simulink model "overall_model"  (R2015a)
settings: Solver=ode45  StartTime=0.0  StopTime=10.0  RelTol=1e-3
libraries: fuzblock x2
settings Model: Creator=BML  LastModifiedBy=BML

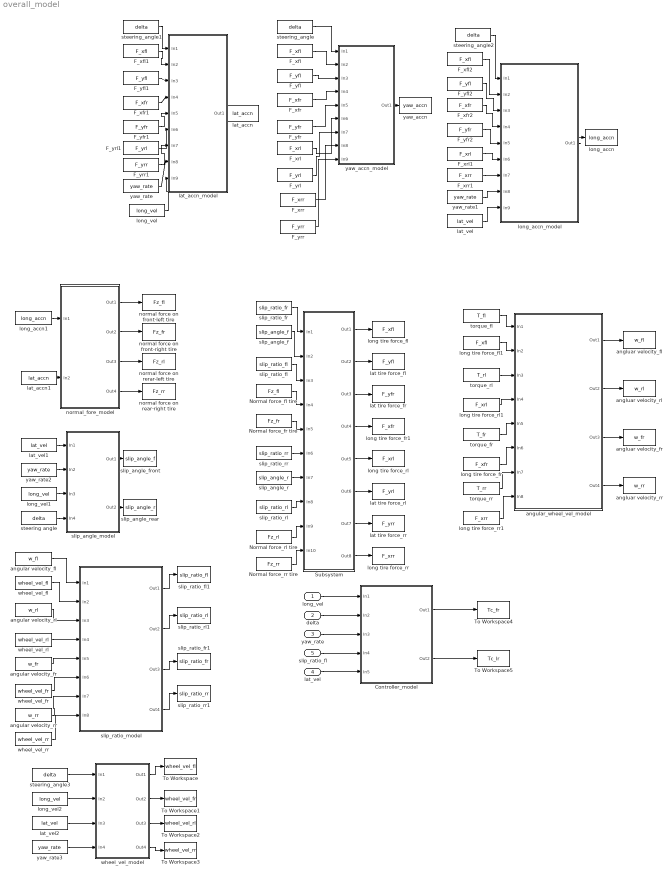
== system overall_model ==
  "  long_vel  " : Inport
  "  delta " : Inport  Port=2
  "  yaw_rate " : Inport  Port=3
  "  lat_vel" : Inport  Port=4
  " slip_ratio_fl  " : Inport  Port=5
  Controller_model : Subsystem
  F_xfl : FromWorkspace  VariableName=F_xfl  SampleTime=0
  F_xfl1 : FromWorkspace  VariableName=F_xfl  SampleTime=0
  F_xfl2 : FromWorkspace  VariableName=F_xfl  SampleTime=0
  F_xfr : FromWorkspace  VariableName=F_xfr  SampleTime=0
  F_xfr1 : FromWorkspace  VariableName=F_xfr  SampleTime=0
  F_xfr2 : FromWorkspace  VariableName=F_xfr  SampleTime=0
  F_xrl : FromWorkspace  VariableName=F_xrl  SampleTime=0
  F_xrl1 : FromWorkspace  VariableName=F_xrl  SampleTime=0
  F_xrr : FromWorkspace  VariableName=F_xrr  SampleTime=0
  F_xrr1 : FromWorkspace  VariableName=F_xrr  SampleTime=0
  F_yfl : FromWorkspace  VariableName=F_yfl  SampleTime=0
  F_yfl1 : FromWorkspace  VariableName=F_yfl  SampleTime=0
  F_yfl2 : FromWorkspace  VariableName=F_yfl  SampleTime=0
  F_yfr : FromWorkspace  VariableName=F_yfr  SampleTime=0
  F_yfr1 : FromWorkspace  VariableName=F_yfr  SampleTime=0
  F_yfr2 : FromWorkspace  VariableName=F_yfr  SampleTime=0
  F_yrl : FromWorkspace  VariableName=F_yrl  SampleTime=0
  F_yrl1 : FromWorkspace  VariableName=F_yrl  SampleTime=0
  F_yrr : FromWorkspace  VariableName=F_yrr  SampleTime=0
  F_yrr1 : FromWorkspace  VariableName=F_yrr  SampleTime=0
  Normal force_fl tire : FromWorkspace  VariableName=Fz_fl  SampleTime=0
  Normal force_fr tire : FromWorkspace  VariableName=Fz_fr  SampleTime=0
  Normal force_rl tire : FromWorkspace  VariableName=Fz_rl  SampleTime=0
  Normal force_rr tire : FromWorkspace  VariableName=Fz_rr  SampleTime=0
  Subsystem : Subsystem
  To Workspace : ToWorkspace  VariableName=wheel_vel_fl  SaveFormat=Timeseries  SampleTime=-1
  To Workspace1 : ToWorkspace  VariableName=wheel_vel_fr  SaveFormat=Timeseries  SampleTime=-1
  To Workspace2 : ToWorkspace  VariableName=wheel_vel_rl  SaveFormat=Timeseries  SampleTime=-1
  To Workspace3 : ToWorkspace  VariableName=wheel_vel_rr  SaveFormat=Timeseries  SampleTime=-1
  To Workspace4 : ToWorkspace  VariableName=Tc_fr  SaveFormat=Timeseries  SampleTime=-1
  To Workspace5 : ToWorkspace  VariableName=Tc_lr  SaveFormat=Timeseries  SampleTime=-1
  angluar velocity_fl : ToWorkspace  VariableName=w_fl  SaveFormat=Timeseries  SampleTime=-1
  angluar velocity_fr : ToWorkspace  VariableName=w_fr  SaveFormat=Timeseries  SampleTime=-1
  angluar velocity_rl : ToWorkspace  VariableName=w_rl  SaveFormat=Timeseries  SampleTime=-1
  angluar velocity_rr : ToWorkspace  VariableName=w_rr  SaveFormat=Timeseries  SampleTime=-1
  angular velocity_fl : FromWorkspace  VariableName=w_fl  SampleTime=0
  angular velocity_fr : FromWorkspace  VariableName=w_fr  SampleTime=0
  angular velocity_rl : FromWorkspace  VariableName=w_rl  SampleTime=0
  angular velocity_rr : FromWorkspace  VariableName=w_rr  SampleTime=0
  angular_wheel_vel_model : Subsystem
  lat tire force_fl : ToWorkspace  VariableName=F_yfl  SaveFormat=Timeseries  SampleTime=-1
  lat tire force_fr : ToWorkspace  VariableName=F_yfr  SaveFormat=Timeseries  SampleTime=-1
  lat tire force_rl : ToWorkspace  VariableName=F_yrl  SaveFormat=Timeseries  SampleTime=-1
  lat tire force_rr : ToWorkspace  VariableName=F_yrr  SaveFormat=Timeseries  SampleTime=-1
  lat_accn : ToWorkspace  VariableName=lat_accn  SaveFormat=Timeseries  SampleTime=-1
  lat_accn1 : FromWorkspace  VariableName=lat_accn  SampleTime=0
  lat_accn_model : Subsystem
  lat_vel : FromWorkspace  VariableName=lat_vel  SampleTime=0
  lat_vel1 : FromWorkspace  VariableName=lat_vel  SampleTime=0
  lat_vel2 : FromWorkspace  VariableName=lat_vel  SampleTime=0
  long tire force_fl : ToWorkspace  VariableName=F_xfl  SaveFormat=Timeseries  SampleTime=-1
  long tire force_fl1 : FromWorkspace  VariableName=F_xfl  SampleTime=0
  long tire force_fr : FromWorkspace  VariableName=F_xfr  SampleTime=0
  long tire force_fr1 : ToWorkspace  VariableName=F_xfr  SaveFormat=Timeseries  SampleTime=-1
  long tire force_rl : ToWorkspace  VariableName=F_xrl  SaveFormat=Timeseries  SampleTime=-1
  long tire force_rl1 : FromWorkspace  VariableName=F_xrl  SampleTime=0
  long tire force_rr : ToWorkspace  VariableName=F_xrr  SaveFormat=Timeseries  SampleTime=-1
  long tire force_rr1 : FromWorkspace  VariableName=F_xrr  SampleTime=0
  long_accn : ToWorkspace  VariableName=long_accn  SaveFormat=Timeseries  SampleTime=-1
  long_accn1 : FromWorkspace  VariableName=long_accn  SampleTime=0
  long_accn_model : Subsystem
  long_vel : FromWorkspace  VariableName=long_vel  SampleTime=0
  long_vel1 : FromWorkspace  VariableName=long_vel  SampleTime=0
  long_vel2 : FromWorkspace  VariableName=long_vel  SampleTime=0
  normal force on front-left tire : ToWorkspace  VariableName=Fz_fl  SaveFormat=Timeseries  SampleTime=-1
  normal force on front-right tire : ToWorkspace  VariableName=Fz_fr  SaveFormat=Timeseries  SampleTime=-1
  normal force on rear-right tire : ToWorkspace  VariableName=Fz_rr  SaveFormat=Timeseries  SampleTime=-1
  normal force on rerar-left tire : ToWorkspace  VariableName=Fz_rl  SaveFormat=Timeseries  SampleTime=-1
  normal_fore_model : Subsystem
  slip_angle_f : FromWorkspace  VariableName=slip_angle_f  SampleTime=0
  slip_angle_front : ToWorkspace  VariableName=slip_angle_f  SaveFormat=Timeseries  SampleTime=-1
  slip_angle_model : Subsystem
  slip_angle_r : FromWorkspace  VariableName=slip_angle_r  SampleTime=0
  slip_angle_rear : ToWorkspace  VariableName=slip_angle_r  SaveFormat=Timeseries  SampleTime=-1
  slip_ratio_fl : FromWorkspace  VariableName=slip_ratio_fl  SampleTime=0
  slip_ratio_fl1 : ToWorkspace  VariableName=slip_ratio_fl  SaveFormat=Timeseries  SampleTime=-1
  slip_ratio_fr : FromWorkspace  VariableName=slip_ratio_fr  SampleTime=0
  slip_ratio_fr1 : ToWorkspace  VariableName=slip_ratio_fr  SaveFormat=Timeseries  SampleTime=-1
  slip_ratio_model : Subsystem
  slip_ratio_rl : FromWorkspace  VariableName=slip_ratio_rl  SampleTime=0
  slip_ratio_rl1 : ToWorkspace  VariableName=slip_ratio_rl  SaveFormat=Timeseries  SampleTime=-1
  slip_ratio_rr : FromWorkspace  VariableName=slip_ratio_rr  SampleTime=0
  slip_ratio_rr1 : ToWorkspace  VariableName=slip_ratio_rr  SaveFormat=Timeseries  SampleTime=-1
  steering angle : FromWorkspace  VariableName=delta  SampleTime=0
  steering_angle{,1..3} (4 alike) : FromWorkspace  VariableName=delta  SampleTime=0
  torque_fl : FromWorkspace  VariableName=T_fl  SampleTime=0
  torque_fr : FromWorkspace  VariableName=T_fr  SampleTime=0
  torque_rl : FromWorkspace  VariableName=T_rl  SampleTime=0
  torque_rr : FromWorkspace  VariableName=T_rr  SampleTime=0
  wheel_vel_fl : FromWorkspace  VariableName=wheel_vel_fl  SampleTime=0
  wheel_vel_fr : FromWorkspace  VariableName=wheel_vel_fr  SampleTime=0
  wheel_vel_model : Subsystem
  wheel_vel_rl : FromWorkspace  VariableName=wheel_vel_rl  SampleTime=0
  wheel_vel_rr : FromWorkspace  VariableName=wheel_vel_rr  SampleTime=0
  yaw_accn : ToWorkspace  VariableName=yaw_accn  SaveFormat=Timeseries  SampleTime=-1
  yaw_accn_model : Subsystem
  yaw_rate{,1..3} (4 alike) : FromWorkspace  VariableName=yaw_rate  SampleTime=0
  wires:
  steering_angle/1 -> yaw_accn_model/1(In1)
  F_xfl/1 -> yaw_accn_model/2(In2)
  F_yfl/1 -> yaw_accn_model/3(In3)
  F_xfr/1 -> yaw_accn_model/4(In4)
  F_yfr/1 -> yaw_accn_model/5(In5)
  F_xrl/1 -> yaw_accn_model/6(In6)
  F_yrl/1 -> yaw_accn_model/7(In7)
  F_xrr/1 -> yaw_accn_model/8(In8)
  F_yrr/1 -> yaw_accn_model/9(In9)
  yaw_accn_model/1(Out1) -> yaw_accn/1
  steering_angle1/1 -> lat_accn_model/1(In1)
  F_xfl1/1 -> lat_accn_model/2(In2)
  F_yfl1/1 -> lat_accn_model/3(In3)
  F_xfr1/1 -> lat_accn_model/4(In4)
  F_yfr1/1 -> lat_accn_model/5(In5)
  F_yrl1/1 -> lat_accn_model/6(In6)
  F_yrr1/1 -> lat_accn_model/7(In7)
  yaw_rate/1 -> lat_accn_model/8(In8)
  long_vel/1 -> lat_accn_model/9(In9)
  lat_accn_model/1(Out1) -> lat_accn/1
  steering_angle2/1 -> long_accn_model/1(In1)
  F_xfl2/1 -> long_accn_model/2(In2)
  F_yfl2/1 -> long_accn_model/3(In3)
  F_xfr2/1 -> long_accn_model/4(In4)
  F_yfr2/1 -> long_accn_model/5(In5)
  F_xrl1/1 -> long_accn_model/6(In6)
  F_xrr1/1 -> long_accn_model/7(In7)
  yaw_rate1/1 -> long_accn_model/8(In8)
  lat_vel/1 -> long_accn_model/9(In9)
  long_accn_model/1(Out1) -> long_accn/1
  long_accn1/1 -> normal_fore_model/1(In1)
  lat_accn1/1 -> normal_fore_model/2(In2)
  normal_fore_model/1(Out1) -> normal force on front-left tire/1
  normal_fore_model/2(Out2) -> normal force on front-right tire/1
  normal_fore_model/3(Out3) -> normal force on rerar-left tire/1
  normal_fore_model/4(Out4) -> normal force on rear-right tire/1
  lat_vel1/1 -> slip_angle_model/1(In1)
  yaw_rate2/1 -> slip_angle_model/2(In2)
  long_vel1/1 -> slip_angle_model/3(In3)
  steering angle/1 -> slip_angle_model/4(In4)
  slip_angle_model/1(Out1) -> slip_angle_front/1
  slip_angle_model/2(Out2) -> slip_angle_rear/1
  angular velocity_fl/1 -> slip_ratio_model/1(In1)
  wheel_vel_fl/1 -> slip_ratio_model/2(In2)
  angular velocity_rl/1 -> slip_ratio_model/3(In3)
  wheel_vel_rl/1 -> slip_ratio_model/4(In4)
  angular velocity_fr/1 -> slip_ratio_model/5(In5)
  wheel_vel_fr/1 -> slip_ratio_model/6(In6)
  angular velocity_rr/1 -> slip_ratio_model/7(In7)
  wheel_vel_rr/1 -> slip_ratio_model/8(In8)
  slip_ratio_model/1(Out1) -> slip_ratio_fl1/1
  slip_ratio_model/2(Out2) -> slip_ratio_rl1/1
  slip_ratio_model/3(Out3) -> slip_ratio_fr1/1
  slip_ratio_model/4(Out4) -> slip_ratio_rr1/1
  steering_angle3/1 -> wheel_vel_model/1(In1)
  long_vel2/1 -> wheel_vel_model/2(In2)
  lat_vel2/1 -> wheel_vel_model/3(In3)
  yaw_rate3/1 -> wheel_vel_model/4(In4)
  wheel_vel_model/1(Out1) -> To Workspace/1
  wheel_vel_model/2(Out2) -> To Workspace1/1
  wheel_vel_model/3(Out3) -> To Workspace2/1
  wheel_vel_model/4(Out4) -> To Workspace3/1
  torque_fl/1 -> angular_wheel_vel_model/1(In1)
  long tire force_fl1/1 -> angular_wheel_vel_model/2(In2)
  torque_rl/1 -> angular_wheel_vel_model/3(In3)
  long tire force_rl1/1 -> angular_wheel_vel_model/4(In4)
  torque_fr/1 -> angular_wheel_vel_model/5(In5)
  long tire force_fr/1 -> angular_wheel_vel_model/6(In6)
  torque_rr/1 -> angular_wheel_vel_model/7(In7)
  long tire force_rr1/1 -> angular_wheel_vel_model/8(In8)
  angular_wheel_vel_model/1(Out1) -> angluar velocity_fl/1
  angular_wheel_vel_model/2(Out2) -> angluar velocity_rl/1
  angular_wheel_vel_model/3(Out3) -> angluar velocity_fr/1
  angular_wheel_vel_model/4(Out4) -> angluar velocity_rr/1
  "  long_vel  "/1 -> Controller_model/1(In1)
  "  delta "/1 -> Controller_model/2(In2)
  "  yaw_rate "/1 -> Controller_model/3(In3)
  " slip_ratio_fl  "/1 -> Controller_model/4(In4)
  "  lat_vel"/1 -> Controller_model/5(In5)
  Controller_model/1(Out1) -> To Workspace4/1
  Controller_model/2(Out2) -> To Workspace5/1
  slip_ratio_fr/1 -> Subsystem/1(In1)
  slip_angle_f/1 -> Subsystem/2(In2)
  slip_ratio_fl/1 -> Subsystem/3(In3)
  Normal force_fl tire/1 -> Subsystem/4(In4)
  Normal force_fr tire/1 -> Subsystem/5(In5)
  slip_ratio_rr/1 -> Subsystem/6(In6)
  slip_angle_r/1 -> Subsystem/7(In7)
  slip_ratio_rl/1 -> Subsystem/8(In8)
  Normal force_rl tire/1 -> Subsystem/9(In9)
  Normal force_rr tire/1 -> Subsystem/10(In10)
  Subsystem/1(Out1) -> long tire force_fl/1
  Subsystem/2(Out2) -> lat tire force_fl/1
  Subsystem/3(Out3) -> lat tire force_fr/1
  Subsystem/4(Out4) -> long tire force_fr1/1
  Subsystem/5(Out5) -> long tire force_rl/1
  Subsystem/6(Out6) -> lat tire force_rl/1
  Subsystem/7(Out7) -> lat tire force_rr/1
  Subsystem/8(Out8) -> long tire force_rr/1

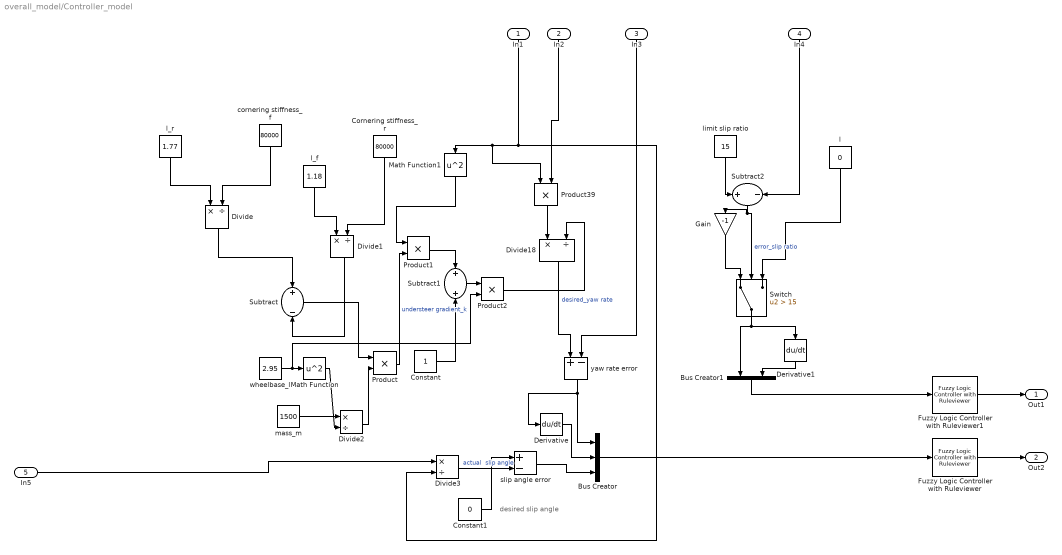
== system overall_model/Controller_model ==
  note: desired
      | slip angle
  In1 : Inport
  In2 : Inport  Port=2
  In3 : Inport  Port=3
  In4 : Inport  Port=4
  In5 : Inport  Port=5
  Bus Creator : BusCreator  Inputs=3
  Bus Creator1 : BusCreator  Inputs=2
  Constant : Constant
  Constant1 : Constant  Value=0
  "Cornering stiffness_r " : Constant  Value=80000
  Derivative : Derivative
  Derivative1 : Derivative
  Divide{,1..3,18} (5 alike) : Product  Inputs=*/
  Fuzzy Logic Controller with Ruleviewer : fuzblock/Fuzzy Logic  Controller  with Ruleviewer  fismatrix=yaw_rate  Ts=2
  Fuzzy Logic Controller with Ruleviewer1 : fuzblock/Fuzzy Logic  Controller  with Ruleviewer  fismatrix=slip_ratio  Ts=2
  Gain : Gain  Gain=-1
  Math Function : Math  Operator=square  SaturateOnIntegerOverflow=on
  Math Function1 : Math  Operator=square  SaturateOnIntegerOverflow=on
  Product{,1..2,39} (4 alike) : Product
  Subtract : Sum  Inputs=+-
  Subtract1 : Sum
  Subtract2 : Sum  Inputs=+-
  Switch : Switch  Criteria=u2 > Threshold  Threshold=15
  "cornering stiffness_f " : Constant  Value=80000
  l : Constant  Value=0
  "l_f " : Constant  Value=1.18
  "l_r " : Constant  Value=1.77
  limit slip ratio : Constant  Value=15
  mass_m : Constant  Value=1500
  "slip angle error  " : Sum  Inputs=+-
  wheelbase_l : Constant  Value=2.95
  "yaw rate error   " : Sum  Inputs=+-
  Out1 : Outport
  Out2 : Outport  Port=2
  wires:
  Fuzzy Logic Controller with Ruleviewer1/1 -> Out1/1
  Divide/1 -> Subtract/1
  Subtract/1 -> Product/1
  Product/1 -> Product1/2  "understeer gradient_k"
  Constant/1 -> Subtract1/2
  Product39/1 -> Divide18/1
  Product2/1 -> Divide18/2
  In2/1 -> Product39/2
  Math Function1/1 -> Product1/1
  Subtract1/1 -> Product2/1
  In5/1 -> Divide3/1
  "l_r "/1 -> Divide/1
  Divide1/1 -> Subtract/2
  "Cornering stiffness_r "/1 -> Divide1/2
  wheelbase_l/1 -> Product2/2, Math Function/1
  mass_m/1 -> Divide2/1
  Math Function/1 -> Divide2/2
  Divide2/1 -> Product/2
  In1/1 -> Divide3/2, Math Function1/1, Product39/1
  "l_f "/1 -> Divide1/1
  "cornering stiffness_f "/1 -> Divide/2
  Product1/1 -> Subtract1/1
  Constant1/1 -> "slip angle error  "/1
  Switch/1 -> Derivative1/1, Bus Creator1/1
  In3/1 -> "yaw rate error   "/2
  Divide18/1 -> "yaw rate error   "/1  "desired_yaw rate"
  Subtract2/1 -> Switch/2, Gain/1  "error_slip ratio"
  Gain/1 -> Switch/1
  "yaw rate error   "/1 -> Bus Creator/1, Derivative/1
  limit slip ratio/1 -> Subtract2/1
  Derivative/1 -> Bus Creator/2
  Bus Creator/1 -> Fuzzy Logic Controller with Ruleviewer/1
  In4/1 -> Subtract2/2
  l/1 -> Switch/3
  Divide3/1 -> "slip angle error  "/2  "actual  slip angle"
  "slip angle error  "/1 -> Bus Creator/3
  Derivative1/1 -> Bus Creator1/2
  Bus Creator1/1 -> Fuzzy Logic Controller with Ruleviewer1/1
  Fuzzy Logic Controller with Ruleviewer/1 -> Out2/1

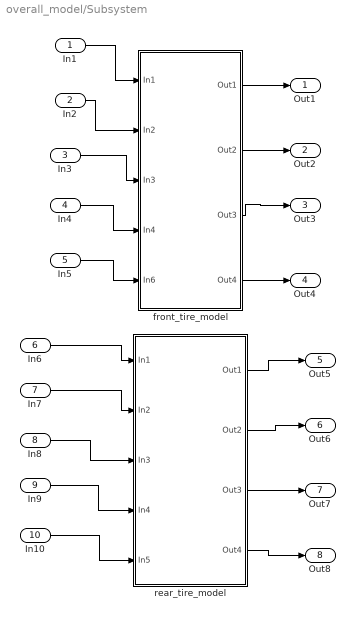
== system overall_model/Subsystem ==
  In1 : Inport
  In2 : Inport  Port=2
  In3 : Inport  Port=3
  In4 : Inport  Port=4
  In5 : Inport  Port=5
  In6 : Inport  Port=6
  In7 : Inport  Port=7
  In8 : Inport  Port=8
  In9 : Inport  Port=9
  In10 : Inport  Port=10
  front_tire_model : Subsystem
  rear_tire_model : Subsystem
  Out1 : Outport
  Out2 : Outport  Port=2
  Out3 : Outport  Port=3
  Out4 : Outport  Port=4
  Out5 : Outport  Port=5
  Out6 : Outport  Port=6
  Out7 : Outport  Port=7
  Out8 : Outport  Port=8
  wires:
  In6/1 -> rear_tire_model/1(In1)
  In7/1 -> rear_tire_model/2(In2)
  rear_tire_model/3(Out3) -> Out7/1
  In8/1 -> rear_tire_model/3(In3)
  rear_tire_model/2(Out2) -> Out6/1
  In10/1 -> rear_tire_model/5(In5)
  rear_tire_model/1(Out1) -> Out5/1
  rear_tire_model/4(Out4) -> Out8/1
  In9/1 -> rear_tire_model/4(In4)
  In2/1 -> front_tire_model/2(In2)
  In1/1 -> front_tire_model/1(In1)
  In3/1 -> front_tire_model/3(In3)
  In5/1 -> front_tire_model/5(In6)
  front_tire_model/1(Out1) -> Out1/1
  front_tire_model/3(Out3) -> Out3/1
  front_tire_model/2(Out2) -> Out2/1
  In4/1 -> front_tire_model/4(In4)
  front_tire_model/4(Out4) -> Out4/1

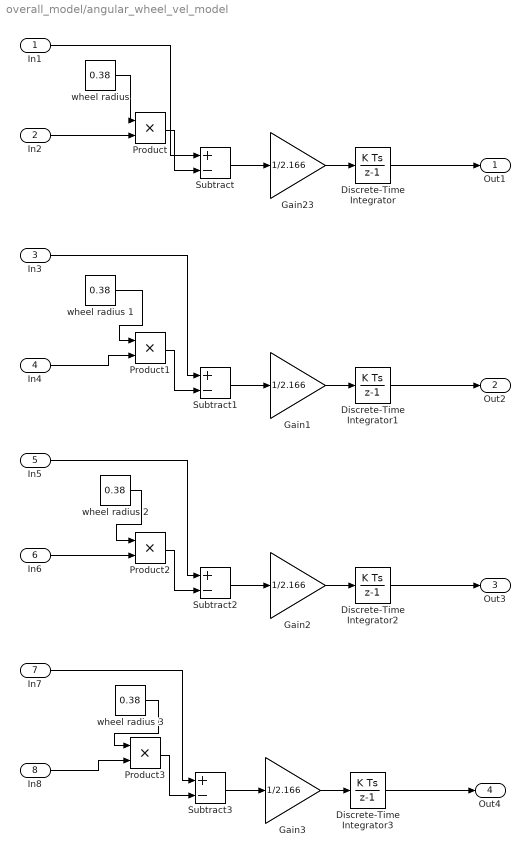
== system overall_model/angular_wheel_vel_model ==
  In1 : Inport
  In2 : Inport  Port=2
  In3 : Inport  Port=3
  In4 : Inport  Port=4
  In5 : Inport  Port=5
  In6 : Inport  Port=6
  In7 : Inport  Port=7
  In8 : Inport  Port=8
  Discrete-Time Integrator{,1..3} (4 alike) : DiscreteIntegrator  InitialConditionSetting=State (most efficient)
  Gain{1..3,23} (4 alike) : Gain  Gain=1/2.166
  Product{,1..3} (4 alike) : Product
  Subtract{,1..3} (4 alike) : Sum  Inputs=+-
  wheel radius {,1..3} (4 alike) : Constant  Value=0.38
  Out1 : Outport
  Out2 : Outport  Port=2
  Out3 : Outport  Port=3
  Out4 : Outport  Port=4
  wires:
  Gain23/1 -> Discrete-Time Integrator/1
  Discrete-Time Integrator/1 -> Out1/1
  In2/1 -> Product/2
  Product/1 -> Subtract/2
  wheel radius 1/1 -> Product1/1
  In3/1 -> Subtract1/1
  In1/1 -> Subtract/1
  Subtract/1 -> Gain23/1
  In4/1 -> Product1/2
  "wheel radius "/1 -> Product/1
  Subtract2/1 -> Gain2/1
  wheel radius 2/1 -> Product2/1
  Product1/1 -> Subtract1/2
  In8/1 -> Product3/2
  In7/1 -> Subtract3/1
  Gain3/1 -> Discrete-Time Integrator3/1
  Subtract1/1 -> Gain1/1
  Gain1/1 -> Discrete-Time Integrator1/1
  Gain2/1 -> Discrete-Time Integrator2/1
  Subtract3/1 -> Gain3/1
  Discrete-Time Integrator3/1 -> Out4/1
  wheel radius 3/1 -> Product3/1
  In6/1 -> Product2/2
  Product3/1 -> Subtract3/2
  In5/1 -> Subtract2/1
  Product2/1 -> Subtract2/2
  Discrete-Time Integrator1/1 -> Out2/1
  Discrete-Time Integrator2/1 -> Out3/1

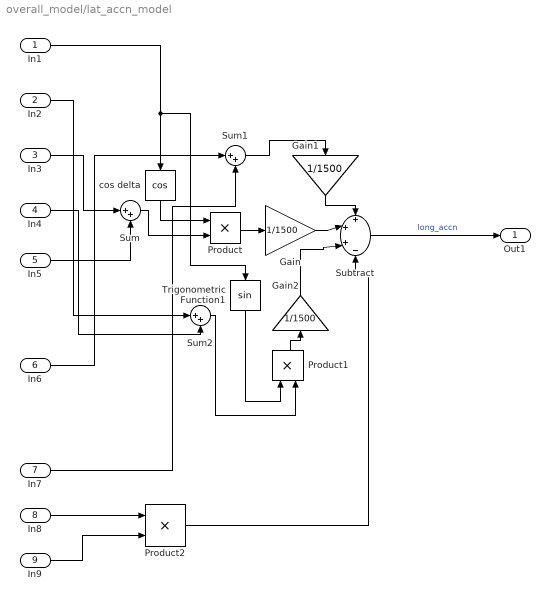
== system overall_model/lat_accn_model ==
  In1 : Inport
  In2 : Inport  Port=2
  In3 : Inport  Port=3
  In4 : Inport  Port=4
  In5 : Inport  Port=5
  In6 : Inport  Port=6
  In7 : Inport  Port=7
  In8 : Inport  Port=8
  In9 : Inport  Port=9
  Gain : Gain  Gain=1/1500
  Gain1 : Gain  Gain=1/1500
  Gain2 : Gain  Gain=1/1500
  Product : Product
  Product1 : Product
  Product2 : Product
  Subtract : Sum  Inputs=+++-
  Sum : Sum  Inputs=|++
  Sum1 : Sum  Inputs=|++
  Sum2 : Sum  Inputs=|++
  Trigonometric Function1 : Trigonometry
  cos delta : Trigonometry  Operator=cos
  Out1 : Outport
  wires:
  Gain/1 -> Subtract/2
  cos delta/1 -> Product/1
  Sum/1 -> Product/2
  Gain1/1 -> Subtract/1
  Sum1/1 -> Gain1/1
  In9/1 -> Product2/2
  Product/1 -> Gain/1
  In1/1 -> Trigonometric Function1/1, cos delta/1
  Trigonometric Function1/1 -> Product1/1
  Sum2/1 -> Product1/2
  Subtract/1 -> Out1/1  "long_accn"
  Product2/1 -> Subtract/4
  Product1/1 -> Gain2/1
  In4/1 -> Sum2/2
  In2/1 -> Sum2/1
  Gain2/1 -> Subtract/3
  In5/1 -> Sum/2
  In6/1 -> Sum1/1
  In8/1 -> Product2/1
  In3/1 -> Sum/1
  In7/1 -> Sum1/2

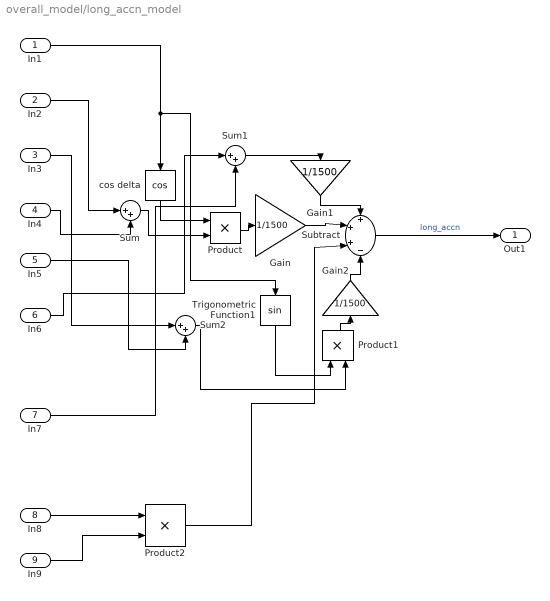
== system overall_model/long_accn_model ==
  In1 : Inport
  In2 : Inport  Port=2
  In3 : Inport  Port=3
  In4 : Inport  Port=4
  In5 : Inport  Port=5
  In6 : Inport  Port=6
  In7 : Inport  Port=7
  In8 : Inport  Port=8
  In9 : Inport  Port=9
  Gain : Gain  Gain=1/1500
  Gain1 : Gain  Gain=1/1500
  Gain2 : Gain  Gain=1/1500
  Product : Product
  Product1 : Product
  Product2 : Product
  Subtract : Sum  Inputs=+++-
  Sum : Sum  Inputs=|++
  Sum1 : Sum  Inputs=|++
  Sum2 : Sum  Inputs=|++
  Trigonometric Function1 : Trigonometry
  cos delta : Trigonometry  Operator=cos
  Out1 : Outport
  wires:
  Product2/1 -> Subtract/3
  Gain/1 -> Subtract/2
  cos delta/1 -> Product/1
  Sum/1 -> Product/2
  Product/1 -> Gain/1
  Gain1/1 -> Subtract/1
  In7/1 -> Sum1/2
  In9/1 -> Product2/2
  Sum1/1 -> Gain1/1
  In4/1 -> Sum/2
  In6/1 -> Sum1/1
  In2/1 -> Sum/1
  In3/1 -> Sum2/1
  In5/1 -> Sum2/2
  Product1/1 -> Gain2/1
  In1/1 -> Trigonometric Function1/1, cos delta/1
  Trigonometric Function1/1 -> Product1/1
  Subtract/1 -> Out1/1  "long_accn"
  Sum2/1 -> Product1/2
  Gain2/1 -> Subtract/4
  In8/1 -> Product2/1

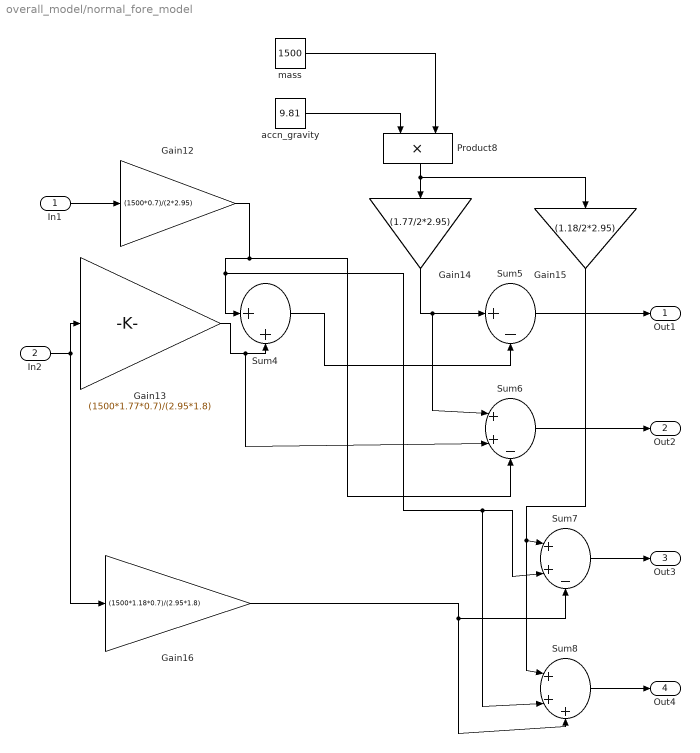
== system overall_model/normal_fore_model ==
  In1 : Inport
  In2 : Inport  Port=2
  Gain12 : Gain  Gain=(1500*0.7)/(2*2.95)
  Gain13 : Gain  Gain=(1500*1.77*0.7)/(2.95*1.8)
  Gain14 : Gain  Gain=(1.77/2*2.95)
  Gain15 : Gain  Gain=(1.18/2*2.95)
  Gain16 : Gain  Gain=(1500*1.18*0.7)/(2.95*1.8)
  Product8 : Product
  Sum4 : Sum  Inputs=|++
  Sum5 : Sum  Inputs=|+-
  Sum6 : Sum  Inputs=|++-
  Sum7 : Sum  Inputs=|++-
  Sum8 : Sum  Inputs=|+++
  "accn_gravity " : Constant  Value=9.81
  mass : Constant  Value=1500
  Out1 : Outport
  Out2 : Outport  Port=2
  Out3 : Outport  Port=3
  Out4 : Outport  Port=4
  wires:
  Gain12/1 -> Sum4/1, Sum8/2, Sum7/2, Sum6/3
  Gain15/1 -> Sum8/1, Sum7/1
  Gain16/1 -> Sum8/3, Sum7/3
  Sum7/1 -> Out3/1
  In2/1 -> Gain13/1, Gain16/1
  Gain13/1 -> Sum6/2, Sum4/2
  Sum5/1 -> Out1/1
  Sum6/1 -> Out2/1
  Sum4/1 -> Sum5/2
  In1/1 -> Gain12/1
  mass/1 -> Product8/2
  Gain14/1 -> Sum5/1, Sum6/1
  Sum8/1 -> Out4/1
  Product8/1 -> Gain14/1, Gain15/1
  "accn_gravity "/1 -> Product8/1

== system overall_model/slip_angle_model ==
  In1 : Inport
  In2 : Inport  Port=2
  In3 : Inport  Port=3
  In4 : Inport  Port=4
  Divide4 : Product  Inputs=*/
  Divide5 : Product  Inputs=*/
  Product : Product
  Product1 : Product
  Sum4 : Sum  Inputs=|++
  Sum5 : Sum  Inputs=|+-
  Sum6 : Sum  Inputs=|+-
  l_f : Constant  Value=1.18
  l_r : Constant  Value=1.77
  Out1 : Outport
  Out2 : Outport  Port=2
  wires:
  In2/1 -> Product1/2, Product/2
  In3/1 -> Divide5/2, Divide4/2
  l_f/1 -> Product/1
  In1/1 -> Sum6/2, Sum4/1
  Divide4/1 -> Sum5/2
  Product/1 -> Sum4/2
  Sum4/1 -> Divide4/1
  Divide5/1 -> Out2/1
  In4/1 -> Sum5/1
  Sum5/1 -> Out1/1
  Product1/1 -> Sum6/1
  l_r/1 -> Product1/1
  Sum6/1 -> Divide5/1

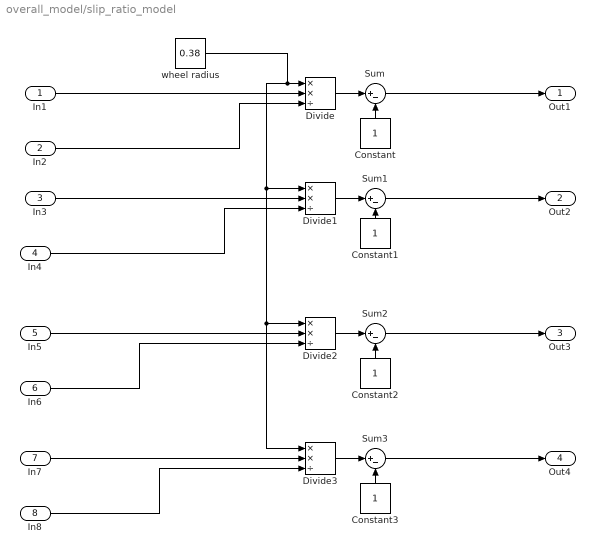
== system overall_model/slip_ratio_model ==
  In1 : Inport
  In2 : Inport  Port=2
  In3 : Inport  Port=3
  In4 : Inport  Port=4
  In5 : Inport  Port=5
  In6 : Inport  Port=6
  In7 : Inport  Port=7
  In8 : Inport  Port=8
  Constant{,1..3} (4 alike) : Constant
  Divide{,1..3} (4 alike) : Product  Inputs=**/
  Sum{,1..3} (4 alike) : Sum  Inputs=|+-
  wheel radius : Constant  Value=0.38
  Out1 : Outport
  Out2 : Outport  Port=2
  Out3 : Outport  Port=3
  Out4 : Outport  Port=4
  wires:
  Constant/1 -> Sum/2
  In1/1 -> Divide/2
  Sum/1 -> Out1/1
  Divide1/1 -> Sum1/1
  Constant1/1 -> Sum1/2
  In3/1 -> Divide1/2
  In2/1 -> Divide/3
  Divide/1 -> Sum/1
  In4/1 -> Divide1/3
  Constant3/1 -> Sum3/2
  In6/1 -> Divide2/3
  In7/1 -> Divide3/2
  In5/1 -> Divide2/2
  In8/1 -> Divide3/3
  Sum1/1 -> Out2/1
  Divide2/1 -> Sum2/1
  Sum2/1 -> Out3/1
  Divide3/1 -> Sum3/1
  Sum3/1 -> Out4/1
  Constant2/1 -> Sum2/2
  wheel radius/1 -> Divide3/1, Divide2/1, Divide1/1, Divide/1

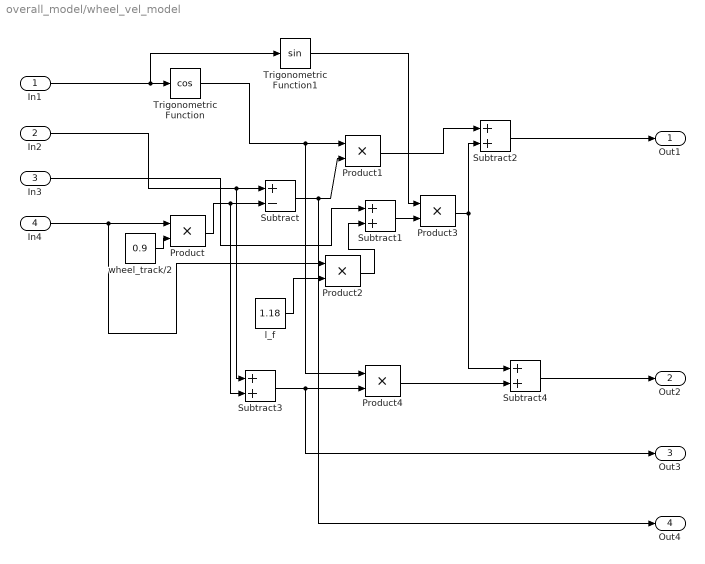
== system overall_model/wheel_vel_model ==
  In1 : Inport
  In2 : Inport  Port=2
  In3 : Inport  Port=3
  In4 : Inport  Port=4
  Product{,1..4} (5 alike) : Product
  Subtract : Sum  Inputs=+-
  Subtract{1..4} (4 alike) : Sum
  Trigonometric Function : Trigonometry  Operator=cos
  Trigonometric Function1 : Trigonometry
  l_f : Constant  Value=1.18
  wheel_track/2 : Constant  Value=0.9
  Out1 : Outport
  Out2 : Outport  Port=2
  Out3 : Outport  Port=3
  Out4 : Outport  Port=4
  wires:
  In2/1 -> Subtract3/1, Subtract/1
  l_f/1 -> Product2/2
  Subtract3/1 -> Out3/1, Product4/2
  Trigonometric Function/1 -> Product4/1, Product1/1
  Subtract1/1 -> Product3/2
  Subtract/1 -> Out4/1, Product1/2
  Product4/1 -> Subtract4/2
  Subtract4/1 -> Out2/1
  In3/1 -> Subtract1/1
  Product/1 -> Subtract3/2, Subtract/2
  Product2/1 -> Subtract1/2
  Product1/1 -> Subtract2/1
  In4/1 -> Product/1, Product2/1
  wheel_track/2/1 -> Product/2
  Trigonometric Function1/1 -> Product3/1
  Subtract2/1 -> Out1/1
  In1/1 -> Trigonometric Function1/1, Trigonometric Function/1
  Product3/1 -> Subtract2/2, Subtract4/1

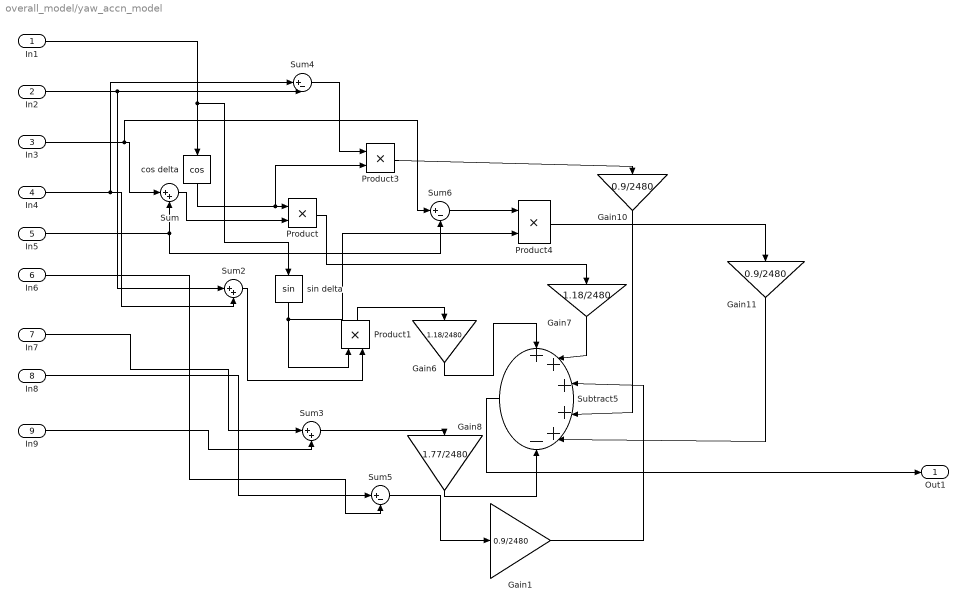
== system overall_model/yaw_accn_model ==
  In1 : Inport
  In2 : Inport  Port=2
  In3 : Inport  Port=3
  In4 : Inport  Port=4
  In5 : Inport  Port=5
  In6 : Inport  Port=6
  In7 : Inport  Port=7
  In8 : Inport  Port=8
  In9 : Inport  Port=9
  Gain1 : Gain  Gain=0.9/2480
  Gain10 : Gain  Gain=0.9/2480
  Gain11 : Gain  Gain=0.9/2480
  Gain6 : Gain  Gain=1.18/2480
  Gain7 : Gain  Gain=1.18/2480
  Gain8 : Gain  Gain=1.77/2480
  Product{,1,3..4} (4 alike) : Product
  Subtract5 : Sum  Inputs=+++++-
  Sum : Sum  Inputs=|++
  Sum2 : Sum  Inputs=|++
  Sum3 : Sum  Inputs=|++
  Sum4 : Sum  Inputs=|+-
  Sum5 : Sum  Inputs=|+-
  Sum6 : Sum  Inputs=|+-
  cos delta : Trigonometry  Operator=cos
  "sin delta " : Trigonometry
  Out1 : Outport
  wires:
  Sum4/1 -> Product3/1
  In1/1 -> "sin delta "/1, cos delta/1
  In7/1 -> Sum3/1
  Product3/1 -> Gain10/1
  Gain10/1 -> Subtract5/4
  In8/1 -> Sum5/1
  In3/1 -> Sum6/1, Sum/1
  Gain11/1 -> Subtract5/5
  In9/1 -> Sum3/2
  In6/1 -> Sum5/2
  "sin delta "/1 -> Product4/2, Product1/1
  cos delta/1 -> Product3/2, Product/1
  Gain7/1 -> Subtract5/2
  In5/1 -> Sum6/2, Sum/2
  Gain6/1 -> Subtract5/1
  Gain8/1 -> Subtract5/6
  Product/1 -> Gain7/1
  In2/1 -> Sum2/1, Sum4/2
  Product1/1 -> Gain6/1
  Sum3/1 -> Gain8/1
  Sum/1 -> Product/2
  Sum2/1 -> Product1/2
  In4/1 -> Sum4/1, Sum2/2
  Sum6/1 -> Product4/1
  Subtract5/1 -> Out1/1
  Sum5/1 -> Gain1/1
  Gain1/1 -> Subtract5/3
  Product4/1 -> Gain11/1

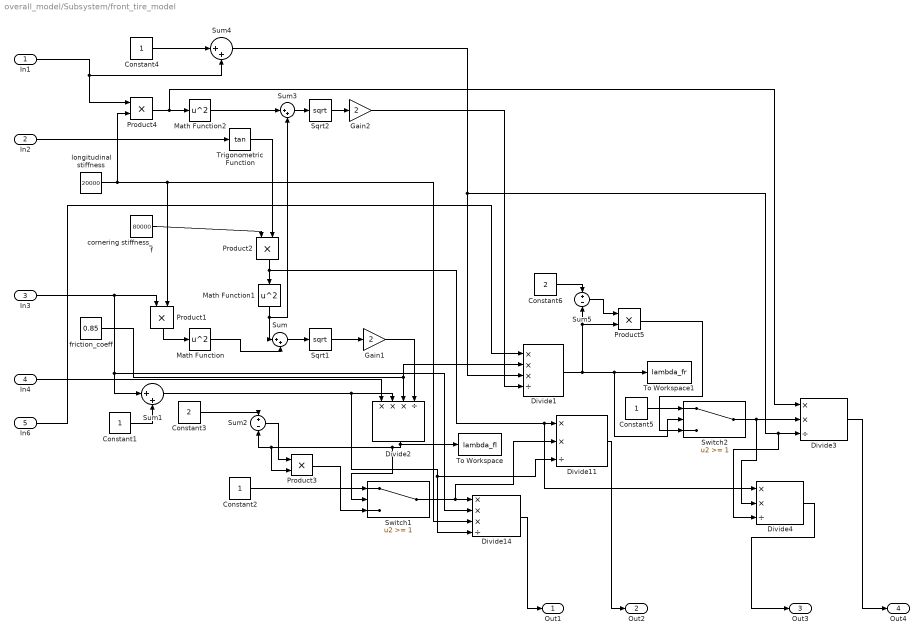
== system overall_model/Subsystem/front_tire_model ==
  In1 : Inport
  In2 : Inport  Port=2
  In3 : Inport  Port=3
  In4 : Inport  Port=4
  In6 : Inport  Port=5
  Constant{1..2,4..5} (4 alike) : Constant
  Constant3 : Constant  Value=2
  Constant6 : Constant  Value=2
  Divide1 : Product  Inputs=***/
  Divide11 : Product  Inputs=**/
  Divide14 : Product  Inputs=***/
  Divide2 : Product  Inputs=***/
  Divide3 : Product  Inputs=**/
  Divide4 : Product  Inputs=**/
  Gain1 : Gain  Gain=2
  Gain2 : Gain  Gain=2
  Math Function : Math  Operator=square  SaturateOnIntegerOverflow=on
  Math Function1 : Math  Operator=square  SaturateOnIntegerOverflow=on
  Math Function2 : Math  Operator=square  SaturateOnIntegerOverflow=on
  Product{1..5} (5 alike) : Product
  Sqrt1 : Sqrt  SaturateOnIntegerOverflow=on
  Sqrt2 : Sqrt  SaturateOnIntegerOverflow=on
  Sum{,1,3..4} (4 alike) : Sum  Inputs=|++
  Sum2 : Sum  Inputs=+-
  Sum5 : Sum  Inputs=+-
  Switch1 : Switch  Threshold=1
  Switch2 : Switch  Threshold=1
  To Workspace : ToWorkspace  VariableName=lambda_fl  SaveFormat=Timeseries  SampleTime=-1
  To Workspace1 : ToWorkspace  VariableName=lambda_fr  SaveFormat=Timeseries  SampleTime=-1
  Trigonometric Function : Trigonometry  Operator=tan
  cornering stiffness_f : Constant  Value=80000
  friction_coeff : Constant  Value=0.85
  longitudinal stiffness : Constant  Value=20000
  Out1 : Outport
  Out2 : Outport  Port=2
  Out3 : Outport  Port=3
  Out4 : Outport  Port=4
  wires:
  Math Function/1 -> Sum/2
  Constant1/1 -> Sum1/2
  Gain1/1 -> Divide2/4
  Trigonometric Function/1 -> Product2/2
  In3/1 -> Divide14/2, Sum1/1, Product1/1
  Sum/1 -> Sqrt1/1
  friction_coeff/1 -> Divide1/2, Divide2/3
  Sqrt1/1 -> Gain1/1
  In4/1 -> Divide2/1
  Product3/1 -> Switch1/3
  Gain2/1 -> Divide1/4
  Math Function1/1 -> Sum3/2, Sum/1
  Sum5/1 -> Product5/1
  Product2/1 -> Divide4/1, Divide11/1, Math Function1/1
  Constant5/1 -> Switch2/1
  cornering stiffness_f/1 -> Product2/1
  Switch2/1 -> Divide4/2, Divide3/2
  Divide14/1 -> Out1/1
  In6/1 -> Divide1/1
  Sum4/1 -> Divide4/3, Divide3/3, Divide1/3
  Constant2/1 -> Switch1/1
  Sum1/1 -> Divide11/3, Divide14/4, Divide2/2
  Divide11/1 -> Out2/1
  In1/1 -> Sum4/2, Product4/1
  Switch1/1 -> Divide11/2, Divide14/1
  Constant4/1 -> Sum4/1
  longitudinal stiffness/1 -> Product4/2, Product1/2, Divide14/3
  Sum3/1 -> Sqrt2/1
  Math Function2/1 -> Sum3/1
  Constant6/1 -> Sum5/1
  Sqrt2/1 -> Gain2/1
  Product4/1 -> Divide3/1, Math Function2/1
  Divide3/1 -> Out4/1
  Divide4/1 -> Out3/1
  Sum2/1 -> Product3/1
  Divide1/1 -> Switch2/2, To Workspace1/1, Sum5/2, Product5/2
  Constant3/1 -> Sum2/1
  Product1/1 -> Math Function/1
  In2/1 -> Trigonometric Function/1
  Divide2/1 -> Switch1/2, Product3/2, Sum2/2, To Workspace/1
  Product5/1 -> Switch2/3

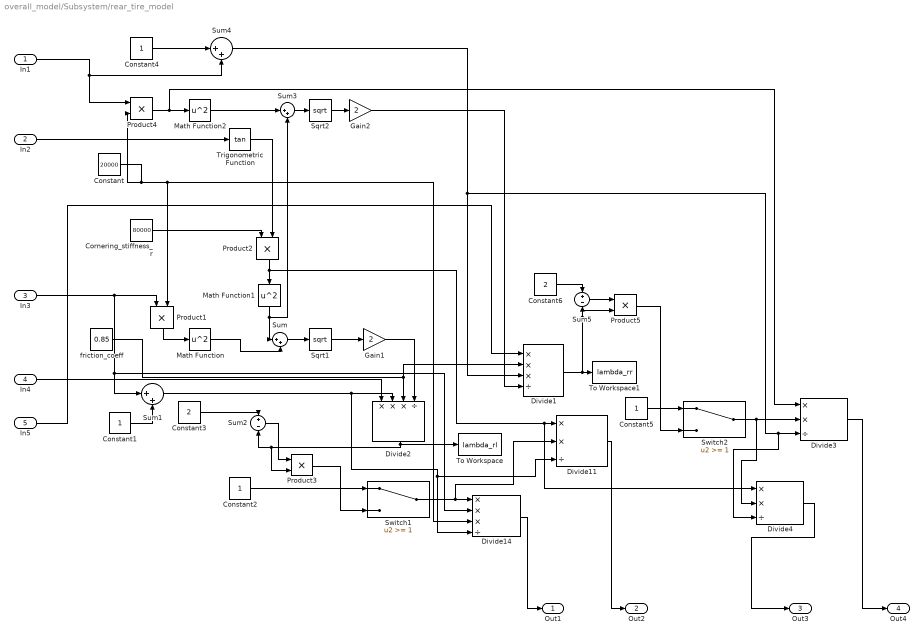
== system overall_model/Subsystem/rear_tire_model ==
  In1 : Inport
  In2 : Inport  Port=2
  In3 : Inport  Port=3
  In4 : Inport  Port=4
  In5 : Inport  Port=5
  Constant : Constant  Value=20000
  Constant{1..2,4..5} (4 alike) : Constant
  Constant3 : Constant  Value=2
  Constant6 : Constant  Value=2
  Cornering_stiffness_r : Constant  Value=80000
  Divide1 : Product  Inputs=***/
  Divide11 : Product  Inputs=**/
  Divide14 : Product  Inputs=***/
  Divide2 : Product  Inputs=***/
  Divide3 : Product  Inputs=**/
  Divide4 : Product  Inputs=**/
  Gain1 : Gain  Gain=2
  Gain2 : Gain  Gain=2
  Math Function : Math  Operator=square  SaturateOnIntegerOverflow=on
  Math Function1 : Math  Operator=square  SaturateOnIntegerOverflow=on
  Math Function2 : Math  Operator=square  SaturateOnIntegerOverflow=on
  Product{1..5} (5 alike) : Product
  Sqrt1 : Sqrt  SaturateOnIntegerOverflow=on
  Sqrt2 : Sqrt  SaturateOnIntegerOverflow=on
  Sum{,1,3..4} (4 alike) : Sum  Inputs=|++
  Sum2 : Sum  Inputs=+-
  Sum5 : Sum  Inputs=+-
  Switch1 : Switch  Threshold=1
  Switch2 : Switch  Threshold=1
  To Workspace : ToWorkspace  VariableName=lambda_rl  SaveFormat=Timeseries  SampleTime=-1
  To Workspace1 : ToWorkspace  VariableName=lambda_rr  SaveFormat=Timeseries  SampleTime=-1
  Trigonometric Function : Trigonometry  Operator=tan
  friction_coeff : Constant  Value=0.85
  Out1 : Outport
  Out2 : Outport  Port=2
  Out3 : Outport  Port=3
  Out4 : Outport  Port=4
  wires:
  Sum2/1 -> Product3/1
  In4/1 -> Divide2/1
  Divide2/1 -> Product3/2, Sum2/2, To Workspace/1
  Product3/1 -> Switch1/3
  Constant3/1 -> Sum2/1
  Constant2/1 -> Switch1/1
  friction_coeff/1 -> Divide1/2, Divide2/3
  Sum1/1 -> Divide11/3, Divide14/4, Divide2/2
  Constant/1 -> Product4/2, Product1/2, Divide14/3
  Divide14/1 -> Out1/1
  Gain1/1 -> Divide2/4
  Constant4/1 -> Sum4/1
  Product2/1 -> Divide4/1, Divide11/1, Math Function1/1
  Sum3/1 -> Sqrt2/1
  Sqrt2/1 -> Gain2/1
  Gain2/1 -> Divide1/4
  In1/1 -> Sum4/2, Product4/1
  Math Function2/1 -> Sum3/1
  Sum5/1 -> Product5/1
  Divide11/1 -> Out2/1
  In5/1 -> Divide1/1
  Math Function1/1 -> Sum3/2, Sum/1
  Cornering_stiffness_r/1 -> Product2/1
  Switch1/1 -> Divide11/2, Divide14/1
  Divide1/1 -> Product5/2, Sum5/2, To Workspace1/1
  Constant6/1 -> Sum5/1
  In3/1 -> Divide14/2, Sum1/1, Product1/1
  Product1/1 -> Math Function/1
  Trigonometric Function/1 -> Product2/2
  Sum/1 -> Sqrt1/1
  Sqrt1/1 -> Gain1/1
  Constant1/1 -> Sum1/2
  In2/1 -> Trigonometric Function/1
  Math Function/1 -> Sum/2
  Constant5/1 -> Switch2/1
  Product4/1 -> Divide3/1, Math Function2/1
  Product5/1 -> Switch2/3
  Switch2/1 -> Divide4/2, Divide3/2
  Divide4/1 -> Out3/1
  Sum4/1 -> Divide4/3, Divide3/3, Divide1/3
  Divide3/1 -> Out4/1
